simulink subsystem "Contolador_BA"  (R2023b)
settings: Solver=VariableStepAuto  StartTime=0.0  StopTime=10.0  RelTol=1e-3
settings Model: Creator=Usuario  LastModifiedBy=Usuario

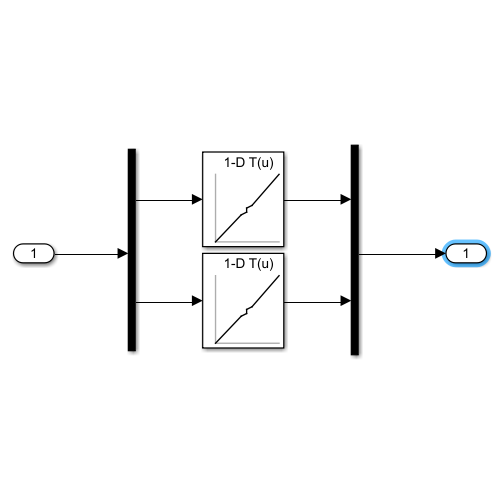
[thumbnail: Simulink's stored preview of the top-level diagram]
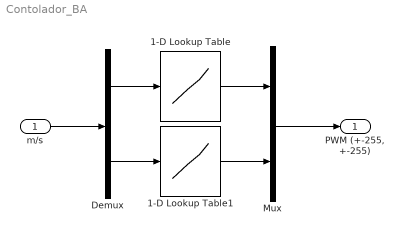
== system Contolador_BA ==
  m/s : Inport
  1-D Lookup Table : Lookup_n-D  NumberOfTableDimensions=1  BreakpointsForDimension1=[-0.483;-0.0845;-1e-05;0;0.0845;0.496]  Table=[-255;-51;-30.6;0;22.95;255]  InternalRulePriority=Speed  RndMeth=Simplest
  1-D Lookup Table1 : Lookup_n-D  NumberOfTableDimensions=1  BreakpointsForDimension1=[-0.502;-0.0845;-1e-05;0;0.0845;0.502]  Table=[-255;-51;-30.6;0;22.95;255]  InternalRulePriority=Speed  RndMeth=Simplest
  Demux : Demux  Outputs=2
  Mux : Mux  Inputs=2
  "PWM (+-255, +-255)" : Outport
  wires:
  m/s/1 -> Demux/1
  Mux/1 -> "PWM (+-255, +-255)"/1
  1-D Lookup Table/1 -> Mux/1
  Demux/1 -> 1-D Lookup Table/1
  Demux/2 -> 1-D Lookup Table1/1
  1-D Lookup Table1/1 -> Mux/2
